simulink model "ExampleProximity"  (Simulink 9.2)
settings: Solver=FixedStepDiscrete  StartTime=0.0  StopTime=60  FixedStep=0.001  RelTol=1e-3  EnableMultiTasking=on
libraries: rFproPhysicsLib x15
settings Model: Creator=enewton  LastModifiedBy=SeanKavanagh  ParamWorkspaceSource=ReferencedWorkspace  TunableVars=LOCAL_PORT_RECV,REMOTE_PORT_RECV,gCGHeight,gFrontTrack,gFrontWheelRadius,gLeftWheelBase,gRearTrack,gRearWheelRadius,gRightWheelBase  TunableVarsStorageClass=Auto,Auto,Auto,Auto,Auto,Auto,Auto,Auto,Auto  TunableVarsTypeQualifier=,,,,,,,,
settings OptimizationCC: DefaultParameterBehavior=Inlined  ExpressionDepthLimit=2147483647
settings DebuggingCC: SolverPrmCheckMsg=warning  InheritedTsInSrcMsg=none  SignalLabelMismatchMsg=error  UnconnectedInputMsg=error  UnconnectedOutputMsg=error  UnconnectedLineMsg=error
settings RTWCC: SystemTargetFile=rfpro.tlc  MakeCommand="make_rtw OPTS=\"-DRUN_PHYSICS\""  TemplateMakefile=rfpro.tmf  Description=rFactor Pro Target (Run Physics)  RetainRTWFile=on  TargetLang=C++
settings STFCustomTargetCC: ModelReferenceCompliant=off  GeneratePreprocessorConditionals=Disable all  CombineOutputUpdateFcns=on  MatFileLogging=on  CPPClassGenCompliant=on  GRTInterface=off  SystemTargetFile=rfpro.tlc
settings GRTTargetCC: ModelReferenceCompliant=off  ParMdlRefBuildCompliant=off  CompOptLevelCompliant=off  ConcurrentExecutionCompliant=off  CombineOutputUpdateFcns=on  GRTInterface=off  UseToolchainInfoCompliant=off  ExtModeMexFile=noextcomm

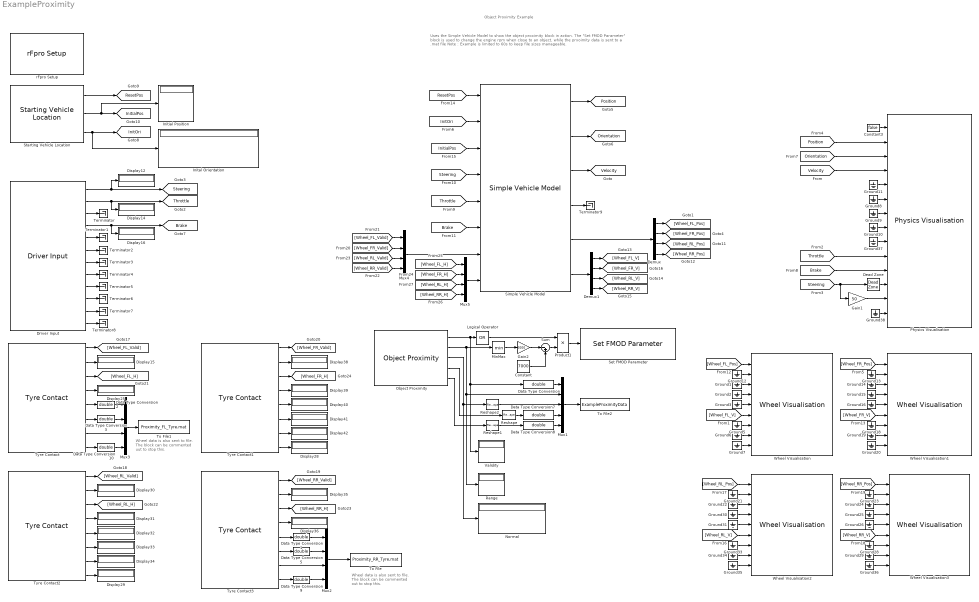
== system ExampleProximity ==
  note: Wheel data is also sent to file.
      | The block can be commented
      | out to stop this.
  note: Object Proximity Example
  note: Uses the Simple Vehicle Model to show the object proximity block in action.
      | The "Set FMOD Parameter" block is used to change the engine rpm when close to an object,
      | while the prxoimity data is sent to a .mat file
      |
      | Note : Example is limited to 60s to keep file sizes manageable.
  note: Wheel data is also sent to file.
      | The block can be commented
      | uut to stop this.
  Constant : Constant  Value=7000
  Constant3 : Constant  Value=false
  Data Type Conversion{,1..3,5,7..10} (9 alike) : DataTypeConversion  OutDataTypeStr=double
  Dead Zone : DeadZone  LowerValue=-0.02  UpperValue=0.02  SaturateOnIntegerOverflow=on
  Demux : Demux
  Demux1 : Demux
  Display{12,14..16,25,28..36,38..42} (19 alike) : Display
  Driver Input : rFproPhysicsLib/Driver Input
  Gain1 : Gain  Gain=50
  Gain2 : Gain  Gain=2000
  Ground{1..3,5..16,18..26,28..31,33..38} (34 alike) : Ground
  Inital Orientation : Display
  Initial Position : Display
  Logical Operator : Logic  Operator=OR  Inputs=1  AllPortsSameDT=off  OutDataTypeStr=boolean
  MinMax : MinMax
  Mux1 : Mux  Inputs=5
  Mux{2..5} (4 alike) : Mux
  Normal : Display
  Object Proximity : rFproPhysicsLib/Object Proximity  offsets=[2.0, 0.5, 0.0; 2.0, -0.5, 0.0]'  rays=[0.0, 3.0, 0.0; 0.0, -3.0, 0.0]'  useReverseByteOrder=off  rFpro__platform=Remote Model - Default
  Physics Visualisation : rFproPhysicsLib/Physics Visualisation  PAR_SKIP_INTERNAL_PHYSICS=off  PAR_ACCEL_VALID=off  PAR_ROT_ACCEL_VALID=off  PAR_GEAR_VALID=off  PAR_RPM_VALID=off  PAR_INPUTS_VALID=on  PAR_STEER_TORQUE_VALID=on  PAR_HEADLIGHTS_ON_VALID=off  PAR_WHEEL_POS_VALID=on  PAR_WHEEL_ORI_VALID=off  PAR_TYRE_PARAMS_VALID=off  PAR_WHEEL_ROTATION_VALID=on  PAR_WHEEL_BRAKE_TEMP_VALID=off  PAR_WHEEL_TREAD_TEMP_VALID=off  PAR_WHEEL_AIR_TEMP_VALID=off  period=-1  offset=0  useReverseByteOrder=on  rFpro__platform=Remote Model - Default
  Product1 : Product  RndMeth=Zero
  Range : Display
  Reshape : Reshape
  Reshape1 : Reshape
  Reshape2 : Reshape
  Set FMOD Parameter : rFproPhysicsLib/Set FMOD Parameter  parameter_name='rpm'  useReverseByteOrder=off  rFpro__platform=Remote Model - Default
  Simple Vehicle Model : rFproPhysicsLib/Internal Utility/Simple Vehicle Model  TIMESTEP=0.001  gCGHeight=0.35  gLeftWheelBase=2.626  gRightWheelBase=2.626  gFrontTrack=1.55  gRearTrack=1.525  gFrontWheelRadius=0.32  gRearWheelRadius=0.33  gWheelDeflection=0
  Starting Vehicle Location : rFproPhysicsLib/Starting Vehicle Location  cg_offset=CG_OFFSET_FROM_NOSE  numPackets=1  rFpro__platform=Remote Model - Default
  Sum : Sum  Inputs=|-+
  Terminator{,1..9} (10 alike) : Terminator
  To File : ToFile  Filename=Proximity_RR_Tyre.mat  MatrixName=RR_Tyre
      settings: Decimation=125
  To File1 : ToFile  Filename=Proximity_FL_Tyre.mat  MatrixName=FL_Tyre
      settings: Decimation=125
  To File2 : ToFile  Filename=ExampleProximityData  MatrixName=ranges
      settings: Decimation=125
  Tyre Contact : rFproPhysicsLib/Tyre Contact  LabelModeActiveChoice=rFproLib_RemoteModel  wheel=FL  contact=[]  radius=0.3  width=0.25  sampleTime=-1  rFpro__platform=Remote Model - Default
  Tyre Contact1 : rFproPhysicsLib/Tyre Contact  LabelModeActiveChoice=rFproLib_RemoteModel  wheel=FR  contact=[]  radius=0.3  width=0.25  sampleTime=-1  rFpro__platform=Remote Model - Default
  Tyre Contact2 : rFproPhysicsLib/Tyre Contact  LabelModeActiveChoice=rFproLib_RemoteModel  wheel=RL  contact=[]  radius=0.3  width=0.25  sampleTime=-1  rFpro__platform=Remote Model - Default
  Tyre Contact3 : rFproPhysicsLib/Tyre Contact  LabelModeActiveChoice=rFproLib_RemoteModel  wheel=RR  contact=[]  radius=0.3  width=0.25  sampleTime=-1  rFpro__platform=Remote Model - Default
  Validity : Display
  Wheel Visualisation : rFproPhysicsLib/Wheel Visualisation  wheelStr=FL
  Wheel Visualisation1 : rFproPhysicsLib/Wheel Visualisation  wheelStr=FR
  Wheel Visualisation2 : rFproPhysicsLib/Wheel Visualisation  wheelStr=RL
  Wheel Visualisation3 : rFproPhysicsLib/Wheel Visualisation  wheelStr=RR
  rFpro Setup : rFproPhysicsLib/rFpro Setup  platform=Remote Model - Default  stopOnSessionEnd=on  usePseudoRealtime=on  syncToRF=on  useReverseByteOrder=off  useRfTime=on  minIterations=4  maxIterations=1000  ipReceiveAddress='127.0.0.1'  ipReceivePort=11054  receiveSampleTime=-1  ipTransmitAddress='127.0.0.1'  ipTransmitPort=11052  transmitSampleTime=-1  pluginType=RUN_PHYSICS  sysTarget=xpctarget.tlc  templateMakeFile=xpc_default_tmf  makeCommand=make_rtw  buildDesc=xPC target
  tag scope: Brake=global, InitOri=global, InitialPos=global, Orientation=global, Position=global, ResetPos=global, Steering=global, Throttle=global, Velocity=global
  wires:
  Constant3/1 -> Physics Visualisation/1
  [Orientation] -> Physics Visualisation/3
  [Velocity] -> Physics Visualisation/4
  [Throttle] -> Physics Visualisation/10
  [Steering] -> Gain1/1, Dead Zone/1
  [Brake] -> Physics Visualisation/11
  Driver Input/1 -> [Steering], Display12/1
  Driver Input/2 -> [Throttle], Display14/1
  Driver Input/4 -> [Brake], Display16/1
  [Position] -> Physics Visualisation/2
  Driver Input/3 -> Terminator/1
  Driver Input/5 -> Terminator1/1
  Driver Input/6 -> Terminator2/1
  Driver Input/7 -> Terminator3/1
  Driver Input/8 -> Terminator4/1
  Driver Input/9 -> Terminator5/1
  Driver Input/10 -> Terminator6/1
  Driver Input/11 -> Terminator7/1
  Driver Input/12 -> Terminator8/1
  Ground8/1 -> Physics Visualisation/6
  Ground9/1 -> Physics Visualisation/7
  Ground10/1 -> Physics Visualisation/8
  Ground11/1 -> Physics Visualisation/5
  Starting Vehicle Location/1 -> [ResetPos]
  Ground1/1 -> Wheel Visualisation/3
  Ground2/1 -> Wheel Visualisation/4
  Ground3/1 -> Wheel Visualisation/5
  Ground5/1 -> Wheel Visualisation/7
  Ground6/1 -> Wheel Visualisation/8
  Ground7/1 -> Wheel Visualisation/9
  Ground12/1 -> Wheel Visualisation/2
  Mux3/1 -> To File1/1
  Data Type Conversion2/1 -> Mux3/1
  Data Type Conversion3/1 -> Mux3/2
  Tyre Contact/7 -> Mux3/3
  Ground13/1 -> Wheel Visualisation1/2
  Ground14/1 -> Wheel Visualisation1/3
  Ground15/1 -> Wheel Visualisation1/4
  Ground16/1 -> Wheel Visualisation1/5
  Ground18/1 -> Wheel Visualisation1/7
  Ground19/1 -> Wheel Visualisation1/8
  Ground20/1 -> Wheel Visualisation1/9
  Ground21/1 -> Wheel Visualisation2/2
  Ground22/1 -> Wheel Visualisation2/3
  Ground30/1 -> Wheel Visualisation2/4
  Ground31/1 -> Wheel Visualisation2/5
  Ground33/1 -> Wheel Visualisation2/7
  Ground34/1 -> Wheel Visualisation2/8
  Ground35/1 -> Wheel Visualisation2/9
  Ground23/1 -> Wheel Visualisation3/2
  Ground24/1 -> Wheel Visualisation3/3
  Ground25/1 -> Wheel Visualisation3/4
  Ground26/1 -> Wheel Visualisation3/5
  Ground28/1 -> Wheel Visualisation3/7
  Ground29/1 -> Wheel Visualisation3/8
  Ground36/1 -> Wheel Visualisation3/9
  Mux2/1 -> To File/1
  Data Type Conversion1/1 -> Mux2/1
  Data Type Conversion5/1 -> Mux2/2
  Tyre Contact3/7 -> Mux2/3
  Starting Vehicle Location/3 -> Inital Orientation/1, [InitOri]
  Starting Vehicle Location/2 -> Initial Position/1, [InitialPos]
  Dead Zone/1 -> Physics Visualisation/12
  Tyre Contact/8 -> Data Type Conversion10/1
  Tyre Contact/6 -> Data Type Conversion3/1
  Tyre Contact/5 -> Data Type Conversion2/1
  Tyre Contact/4 -> Display25/1
  Tyre Contact/1 -> [Wheel_FL_Valid]
  Tyre Contact/2 -> Display15/1
  Tyre Contact1/8 -> Display28/1
  Tyre Contact1/7 -> Display42/1
  Tyre Contact1/6 -> Display41/1
  Tyre Contact1/5 -> Display40/1
  Tyre Contact1/4 -> Display39/1
  Tyre Contact1/1 -> [Wheel_FR_Valid]
  Tyre Contact1/2 -> Display38/1
  Tyre Contact2/8 -> Display29/1
  Tyre Contact2/7 -> Display34/1
  Tyre Contact2/6 -> Display33/1
  Tyre Contact2/5 -> Display32/1
  Tyre Contact2/4 -> Display31/1
  Tyre Contact2/1 -> [Wheel_RL_Valid]
  Tyre Contact2/2 -> Display30/1
  Tyre Contact3/8 -> Data Type Conversion9/1
  Tyre Contact3/6 -> Data Type Conversion5/1
  Tyre Contact3/5 -> Data Type Conversion1/1
  Tyre Contact3/4 -> Display36/1
  Tyre Contact3/1 -> [Wheel_RR_Valid]
  Tyre Contact3/2 -> Display35/1
  Object Proximity/5 -> Reshape1/1
  Object Proximity/4 -> Reshape/1
  Object Proximity/3 -> Normal/1, Reshape2/1
  Object Proximity/2 -> MinMax/1, Range/1, Mux1/2
  MinMax/1 -> Gain2/1
  Constant/1 -> Sum/2
  Gain2/1 -> Sum/1
  Sum/1 -> Product1/2
  Object Proximity/1 -> Logical Operator/1, Validity/1, Data Type Conversion/1
  Logical Operator/1 -> Product1/1
  Product1/1 -> Set FMOD Parameter/1
  Mux1/1 -> To File2/1
  Data Type Conversion/1 -> Mux1/1
  Reshape/1 -> Data Type Conversion7/1
  Reshape1/1 -> Data Type Conversion8/1
  Reshape2/1 -> Mux1/3
  Data Type Conversion7/1 -> Mux1/4
  Data Type Conversion8/1 -> Mux1/5
  [Wheel_RL_Valid] -> Mux4/3
  [Wheel_RR_Valid] -> Mux4/4
  [Wheel_FR_Valid] -> Mux4/2
  [Wheel_FR_H] -> Mux5/2
  [Wheel_FL_H] -> Mux5/1
  [Wheel_RR_H] -> Mux5/4
  [Wheel_RL_H] -> Mux5/3
  Mux4/1 -> Simple Vehicle Model/7
  Demux1/1 -> [Wheel_FL_V]
  Demux1/2 -> [Wheel_FR_V]
  Demux1/3 -> [Wheel_RL_V]
  Demux1/4 -> [Wheel_RR_V]
  Simple Vehicle Model/6 -> Demux1/1
  Simple Vehicle Model/5 -> Demux/1
  Demux/1 -> [Wheel_FL_Pos]
  Demux/2 -> [Wheel_FR_Pos]
  Demux/3 -> [Wheel_RL_Pos]
  Demux/4 -> [Wheel_RR_Pos]
  Simple Vehicle Model/1 -> [Position]
  Simple Vehicle Model/2 -> [Orientation]
  Simple Vehicle Model/3 -> [Velocity]
  [Wheel_FL_Valid] -> Mux4/1
  Mux5/1 -> Simple Vehicle Model/8
  [InitialPos] -> Simple Vehicle Model/3
  [Steering] -> Simple Vehicle Model/4
  [Throttle] -> Simple Vehicle Model/5
  [Brake] -> Simple Vehicle Model/6
  [ResetPos] -> Simple Vehicle Model/1
  [Wheel_FL_Pos] -> Wheel Visualisation/1
  [Wheel_FR_Pos] -> Wheel Visualisation1/1
  [Wheel_RL_Pos] -> Wheel Visualisation2/1
  [Wheel_RR_Pos] -> Wheel Visualisation3/1
  Ground37/1 -> Physics Visualisation/9
  Ground38/1 -> Physics Visualisation/14
  [Wheel_RR_V] -> Wheel Visualisation3/6
  [Wheel_FR_V] -> Wheel Visualisation1/6
  [Wheel_FL_V] -> Wheel Visualisation/6
  [Wheel_RL_V] -> Wheel Visualisation2/6
  Tyre Contact1/3 -> [Wheel_FR_H]
  Tyre Contact/3 -> [Wheel_FL_H]
  Tyre Contact2/3 -> [Wheel_RL_H]
  Tyre Contact3/3 -> [Wheel_RR_H]
  [InitOri] -> Simple Vehicle Model/2
  Data Type Conversion9/1 -> Mux2/4
  Data Type Conversion10/1 -> Mux3/4
  Gain1/1 -> Physics Visualisation/13
  Simple Vehicle Model/4 -> Terminator9/1
